simulink model "D5"  (R2019b)
settings: Solver=ode8  StartTime=0.0  StopTime=2  FixedStep=0.001000  RelTol=1e-3
settings Model: Creator=nahkusaidy  LastModifiedBy=nahkusaidy

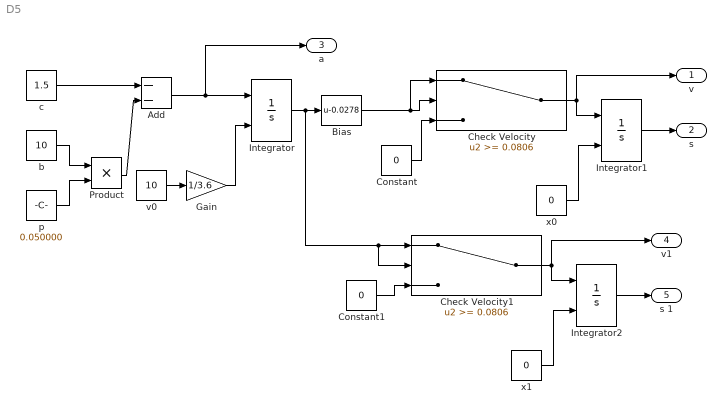
== system D5 ==
  Add : Sum  Inputs=--
  Bias : Bias  Bias=-0.0278
  Check Velocity : Switch  Threshold=0.0806
  Check Velocity1 : Switch  Threshold=0.0806
  Constant : Constant  Value=0
  Constant1 : Constant  Value=0
  Gain : Gain  Gain=1/3.6
  Integrator : Integrator  InitialConditionSource=external
  Integrator1 : Integrator  InitialConditionSource=external
  Integrator2 : Integrator  InitialConditionSource=external
  Product : Product
  b : Constant  Value=10
  c : Constant  Value=1.5
  p : Constant  Value=0.050000
  v0 : Constant  Value=10
  x0 : Constant  Value=0
  x1 : Constant  Value=0
  v : Outport
  "s " : Outport  Port=2
  a : Outport  Port=3
  v1 : Outport  Port=4
  s 1 : Outport  Port=5
  wires:
  c/1 -> Add/1
  b/1 -> Product/1
  p/1 -> Product/2
  Product/1 -> Add/2
  Integrator1/1 -> "s "/1
  x0/1 -> Integrator1/2
  v0/1 -> Gain/1
  Gain/1 -> Integrator/2
  Constant/1 -> Check Velocity/3
  Check Velocity/1 -> Integrator1/1, v/1
  Add/1 -> Integrator/1, a/1
  Bias/1 -> Check Velocity/1, Check Velocity/2
  Integrator/1 -> Check Velocity1/2, Check Velocity1/1, Bias/1
  Integrator2/1 -> s 1/1
  x1/1 -> Integrator2/2
  Check Velocity1/1 -> Integrator2/1, v1/1
  Constant1/1 -> Check Velocity1/3
